simulink model "CornerDetectionHDL_Matlab_Default"  (R2017b)
settings: Solver=FixedStepDiscrete  StartTime=0.0  StopTime=simTime  RelTol=1e-3
InitFcn:
  | % block settings for 240p, change format as appropriate
  | frm2pix = visionhdl.FrameToPixels;
  | frm2pix.VideoFormat = '240p';
  | [activePixelsPerLine, activeLines, totalPixels] = getparamfromfrm2pix(frm2pix);
  | numFrames = 100;
  | simTime = numFrames;
  | % pixel control bus
  | evalin('base','pixelcontrolbus');
undefined symbols (not defined in the file): fspecial, gray, Rec, SDTV
libraries: visionhdlfilter x5, simulink x3, visionhdlio x2, visionconversions x1, visionanalysis x1, visionhdlutilities x1, visionhdlconversions x1, visionhdlmisc x1
settings Model: DataTypeOverride=Off  Creator=The MathWorks, Inc.  LastModifiedBy=KAU-Sprinter
settings DataIOCC: LimitDataPoints=on  SaveFormat=Array  SaveOutput=off  SignalLogging=off  SaveTime=off
settings OptimizationCC: BlockReduction=off  ConditionallyExecuteInputs=off  DefaultParameterBehavior=Inlined  LifeSpan=inf
settings DebuggingCC: AlgebraicLoopMsg=error  ArtificialAlgebraicLoopMsg=none  SingleTaskRateTransMsg=error  IntegerOverflowMsg=none  ParameterPrecisionLossMsg=none  AllowSymbolicDim=off  StrictBusMsg=ErrorOnBusTreatedAsVector  SFUnexpectedBacktrackingDiag=warning  SFNoUnconditionalDefaultTransitionDiag=warning  SFExecutionAtInitializationDiag=none  IntegerSaturationMsg=none
settings HardwareCC: ProdBitPerPointer=32  ProdBitPerSizeT=32  ProdBitPerPtrDiffT=32  ProdLargestAtomicFloat=None  ProdIntDivRoundTo=Undefined  ProdEndianess=Unspecified  ProdWordSize=32  ProdHWDeviceType=ASIC/FPGA->ASIC/FPGA  ProdEqTarget=off
settings ModelReferenceCC: PropagateSignalLabelsOutOfModel=off
settings CodeAppCC: StateflowObjectComments=on
settings GRTTargetCC: TargetLangStandard=C89/C90 (ANSI)  GeneratePreprocessorConditionals=Disable all
settings ConfigComp: CovMetricSettings=dw  CovHtmlReporting=on  CovSaveCumulativeToWorkspaceVar=on  CovSaveSingleToWorkspaceVar=on  CovExternalEMLEnable=off  CovSFcnEnable=off

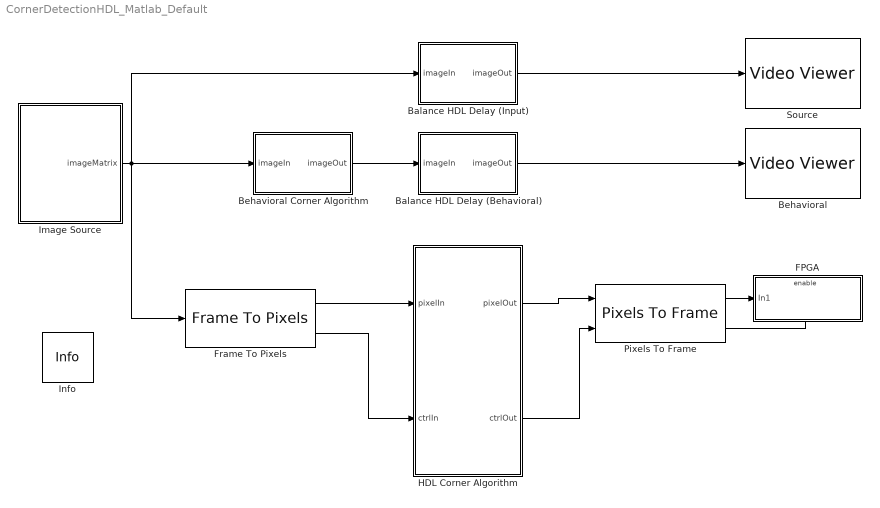
== system CornerDetectionHDL_Matlab_Default ==
  Balance HDL Delay (Behavioral) : Subsystem
  Balance HDL Delay (Input) : Subsystem
  Behavioral : VideoViewer  FigPos=[400.2 479.6 410.4 300]
  Behavioral Corner Algorithm : Subsystem
  FPGA : Subsystem
  Frame To Pixels : visionhdlio/Frame To Pixels  NumComponents=3  VideoFormat=240p  ActivePixelsPerLine=32  ActiveVideoLines=18  TotalPixelsPerLine=42  TotalVideoLines=28  StartingActiveLine=6  FrontPorch=5  SampleTime=0
      settings: SourceProductName=Vision HDL Toolbox  SourceProductBaseCode=VT
  HDL Corner Algorithm : Subsystem  TreatAsAtomicUnit=on
  Image Source : Subsystem  mask(Panning Video Source){VideoFormat=240p}
      mask prompts: VideoFormat "Video Format"
      mask TypeOptions VideoFormat: 240p | 480p | 1080p | Custom
      mask Callback VideoFormat:
      | blk = gcb;
      | set_param(blk,'MaskSelfModifiable','on');
      | maskStr = get_param(blk,'MaskValues');
      | 
      | if strcmpi(maskStr{1},'Custom')
      |     set_param([blk,'/Lines'],'Value',sprintf('[1:%d]',18));
      |     set_param([blk,'/Pixels'],'Value',sprintf('[1:%d]',32));
      | elseif strcmpi(maskStr{1},'240p')
      |     set_param([blk,'/Lines'],'Value',sprintf('[1:%d]',240));
      |     set_param([blk,'/Pixels'],'Value',sprintf('[1:%d]',320));
      | elseif strcmpi(maskStr{1},'480p')
      |     set_param([blk,'/Lines'],'Value',sprintf('[1:%d]',480));
      |     set_param([blk,'/Pixels'],'Value',sprintf('[1:%d]',640));
      | else
      |     set_param([blk,'/Lines'],'Value',sprintf('[1:%d]',1080));
      |     set_param([blk,'/Pixels'],'Value',sprintf('[1:%d]',1920));
      | end
      mask Display: image('cornerboxes.png')
  Info : visionhdlmisc/Info  SystemSampleTime=-1
      settings: SourceProductName=Vision HDL Toolbox  SourceProductBaseCode=VT
  Pixels To Frame : visionhdlio/Pixels To Frame  NumComponents=3  VideoFormat=240p  ActivePixelsPerLine=32  ActiveVideoLines=18  TotalPixelsPerLine=42  TotalVideoLines=28
      settings: SourceProductName=Vision HDL Toolbox  SourceProductBaseCode=VT
  Source : VideoViewer  FigPos=[12.2 436.4 409.6 300]
  wires:
  Image Source/1(imageMatrix) -> Balance HDL Delay (Input)/1(imageIn), Frame To Pixels/1, Behavioral Corner Algorithm/1(imageIn)
  Behavioral Corner Algorithm/1(imageOut) -> Balance HDL Delay (Behavioral)/1(imageIn)
  Frame To Pixels/1 -> HDL Corner Algorithm/1(pixelIn)
  Frame To Pixels/2 -> HDL Corner Algorithm/2(ctrlIn)
  Pixels To Frame/2 -> FPGA/Enable
  Pixels To Frame/1 -> FPGA/1(In1)
  HDL Corner Algorithm/1(pixelOut) -> Pixels To Frame/1
  HDL Corner Algorithm/2(ctrlOut) -> Pixels To Frame/2
  Balance HDL Delay (Input)/1(imageOut) -> Source/1
  Balance HDL Delay (Behavioral)/1(imageOut) -> Behavioral/1

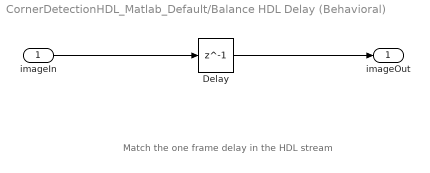
== system CornerDetectionHDL_Matlab_Default/Balance HDL Delay (Behavioral) ==
  note: Match the one frame delay in the HDL stream
  imageIn : Inport
  Delay : Delay  DelayLength=1
  imageOut : Outport
  wires:
  Delay/1 -> imageOut/1
  imageIn/1 -> Delay/1

== system CornerDetectionHDL_Matlab_Default/Balance HDL Delay (Input) ==
  note: Match the one frame delay in the HDL stream
  imageIn : Inport
  Delay : Delay  DelayLength=1
  imageOut : Outport
  wires:
  imageIn/1 -> Delay/1
  Delay/1 -> imageOut/1

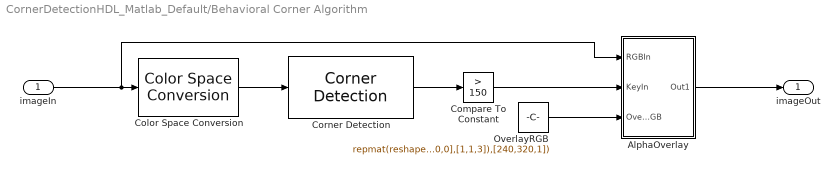
== system CornerDetectionHDL_Matlab_Default/Behavioral Corner Algorithm ==
  imageIn : Inport
  AlphaOverlay : Subsystem
  Color Space Conversion : visionconversions/Color Space  Conversion  conversion=Obsolete  conversionActive=R'G'B' to intensity  wp_str=D65  rec=Rec. 601 (SDTV)  sys=1125/60/2:1  imagePorts=One multidimensional signal
      settings: SourceProductName=Computer Vision System Toolbox
  Compare To Constant : simulink/Logic and Bit Operations/Compare To Constant  relop=>  const=150  OutDataTypeStr=boolean
  Corner Detection : visionanalysis/Corner Detection  method=Harris corner detection (Harris & Stephens)  factor=0.04  filter=fspecial('gaussian', [1 5], 1.5)  thrInten=0.1  thrAngle=157.5  output=Obsolete9b  outputInUse=Metric matrix  maxNum=200  thrMetric=0.0005  neighborSize=[11 11]  isOutVarDim=on  accumMode=Binary point scaling  accumWordLength=32  accumFracLength=0  prodOutputMode=Binary point scaling  prodOutputWordLength=32  prodOutputFracLength=0  memoryMode=Binary point scaling  memoryWordLength=32  memoryFracLength=0  firstCoeffMode=Specify word length  firstCoeffWordLength=16  firstCoeffFracLength=16  roundingMode=Floor  overflowMode=off
      settings: SourceProductName=Computer Vision System Toolbox  SourceProductBaseCode=VP
  "OverlayRGB " : Constant  Value=repmat(reshape([255,0,0],[1,1,3]),[240,320,1])  OutDataTypeStr=uint8
  imageOut : Outport
  wires:
  imageIn/1 -> AlphaOverlay/1(RGBIn), Color Space Conversion/1
  Corner Detection/1 -> Compare To Constant/1
  Color Space Conversion/1 -> Corner Detection/1
  Compare To Constant/1 -> AlphaOverlay/2(KeyIn)
  AlphaOverlay/1(Out1) -> imageOut/1
  "OverlayRGB "/1 -> AlphaOverlay/3(OverlayRGB)

== system CornerDetectionHDL_Matlab_Default/FPGA ==
  In1 : Inport
  Enable : EnablePort
  FPGA Video : VideoViewer  colormapValue=gray(256)  FigPos=[864.2 436.4 416 298.4]
  wires:
  In1/1 -> FPGA Video/1

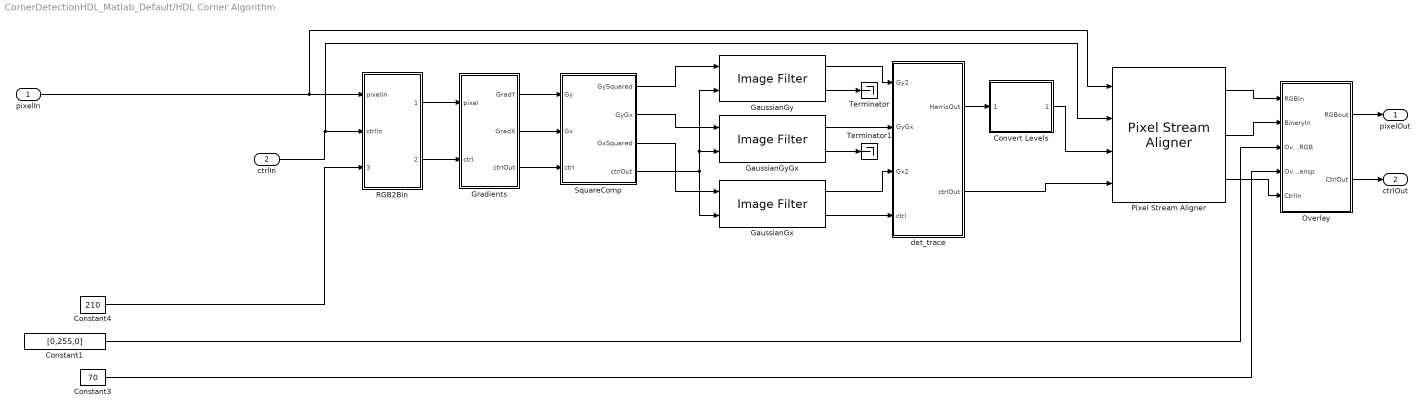
== system CornerDetectionHDL_Matlab_Default/HDL Corner Algorithm ==
  pixelIn : Inport
  ctrlIn : Inport  Port=2
  Constant1 : Constant  Value=[0,255,0]  VectorParams1D=off  OutDataTypeStr=uint8  SampleTime=-1
  Constant3 : Constant  Value=70  OutDataTypeStr=uint8  SampleTime=-1
  Constant4 : Constant  Value=210  OutDataTypeStr=uint8  SampleTime=-1
  Convert Levels : Subsystem
  GaussianGx : visionhdlfilter/Image Filter  Coefficients=fspecial('gaussian',[5,5],1.5)  PaddingMethod=Constant  PaddingValue=0  LineBufferSize=2048  SimulateUsing=Code generation  roundingMode=Floor  overflowMode=off  CoeffDataTypeStr=fixdt(1,18,21)  CoeffMin=[]  CoeffMax=[]  OutputMin=[]  OutputMax=[]
      settings: SourceProductName=Vision HDL Toolbox  SourceProductBaseCode=VT
  GaussianGy : visionhdlfilter/Image Filter  Coefficients=fspecial('gaussian',[5,5],1.5)  PaddingMethod=Constant  PaddingValue=0  LineBufferSize=2048  SimulateUsing=Code generation  roundingMode=Floor  overflowMode=off  CoeffDataTypeStr=fixdt(1,18,21)  CoeffMin=[]  CoeffMax=[]  OutputMin=[]  OutputMax=[]
      settings: SourceProductName=Vision HDL Toolbox  SourceProductBaseCode=VT
  GaussianGyGx : visionhdlfilter/Image Filter  Coefficients=fspecial('gaussian',[5,5],1.5)  PaddingMethod=Constant  PaddingValue=0  LineBufferSize=2048  SimulateUsing=Code generation  roundingMode=Floor  overflowMode=off  CoeffDataTypeStr=fixdt(1,18,21)  CoeffMin=[]  CoeffMax=[]  OutputMin=[]  OutputMax=[]
      settings: SourceProductName=Vision HDL Toolbox  SourceProductBaseCode=VT
  Gradients : Subsystem
  Overlay : Subsystem
  Pixel Stream Aligner : visionhdlutilities/Pixel Stream Aligner  LineBufferSize=2048  MaximumNumberOfLines=10  SimulateUsing=Code generation
      settings: SourceProductName=Vision HDL Toolbox  SourceProductBaseCode=VT
  RGB2Bin : Subsystem
  SquareComp : Subsystem
  Terminator : Terminator
  Terminator1 : Terminator
  det_trace : Subsystem
  pixelOut : Outport
  ctrlOut : Outport  Port=2
  wires:
  Constant1/1 -> Overlay/3(OverlayRGB)
  Constant4/1 -> RGB2Bin/3(SliceLevel)
  RGB2Bin/2(ctrlOut) -> Gradients/2(ctrl)
  Overlay/2("CtrlOut ") -> ctrlOut/1
  Convert Levels/1(PixelOut) -> Pixel Stream Aligner/3
  RGB2Bin/1(pixelOut) -> Gradients/1(pixel)
  Overlay/1(RGBout) -> pixelOut/1
  det_trace/1(HarrisOut) -> Convert Levels/1(HarrisIn)
  Constant3/1 -> Overlay/4(OverlayTransp)
  det_trace/2(ctrlOut) -> Pixel Stream Aligner/4
  Gradients/3(ctrlOut) -> SquareComp/3(ctrl)
  Gradients/2(GradX) -> SquareComp/2(Gx)
  Gradients/1(GradY) -> SquareComp/1(Gy)
  ctrlIn/1 -> Pixel Stream Aligner/2, RGB2Bin/2(ctrlIn)
  pixelIn/1 -> Pixel Stream Aligner/1, RGB2Bin/1(pixelIn)
  GaussianGx/2 -> det_trace/4(ctrl)
  GaussianGx/1 -> det_trace/3(Gx2)
  GaussianGyGx/1 -> det_trace/2(GyGx)
  GaussianGy/1 -> det_trace/1(Gy2)
  SquareComp/3(GxSquared) -> GaussianGx/1
  SquareComp/2(GyGx) -> GaussianGyGx/1
  SquareComp/1(GySquared) -> GaussianGy/1
  SquareComp/4(ctrlOut) -> GaussianGx/2, GaussianGy/2, GaussianGyGx/2
  GaussianGyGx/2 -> Terminator1/1
  GaussianGy/2 -> Terminator/1
  Pixel Stream Aligner/1 -> Overlay/1(RGBIn)
  Pixel Stream Aligner/2 -> Overlay/2(BinaryIn)
  Pixel Stream Aligner/3 -> Overlay/5(CtrlIn)

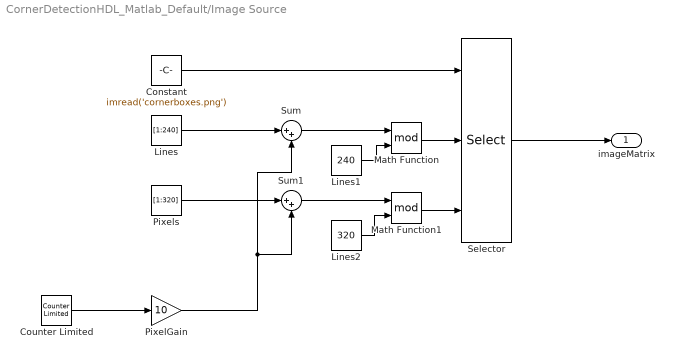
== system CornerDetectionHDL_Matlab_Default/Image Source ==
  Constant : Constant  Value=imread('cornerboxes.png')  VectorParams1D=off
  Counter Limited : simulink/Sources/Counter Limited  uplimit=100  tsamp=1
  Lines : Constant  Value=[1:240]
  Lines1 : Constant  Value=240
  Lines2 : Constant  Value=320
  Math Function : Math  Operator=mod  SaturateOnIntegerOverflow=on
  Math Function1 : Math  Operator=mod  SaturateOnIntegerOverflow=on
  PixelGain : Gain  Gain=10  OutDataTypeStr=double
  Pixels : Constant  Value=[1:320]
  Selector : Selector  NumberOfDimensions=3  IndexMode=Zero-based  InputPortWidth=3  IndexOptions=Index vector (port),Index vector (port),Select all  Indices=[1 3],1,1  OutputSizes=1,1,1
  Sum : Sum  Inputs=|++
  Sum1 : Sum  Inputs=|++
  imageMatrix : Outport
  wires:
  Counter Limited/1 -> PixelGain/1
  Selector/1 -> imageMatrix/1
  Math Function1/1 -> Selector/3
  Constant/1 -> Selector/1
  Math Function/1 -> Selector/2
  Sum/1 -> Math Function/1
  Lines/1 -> Sum/1
  Pixels/1 -> Sum1/1
  PixelGain/1 -> Sum1/2, Sum/2
  Lines1/1 -> Math Function/2
  Lines2/1 -> Math Function1/2
  Sum1/1 -> Math Function1/1

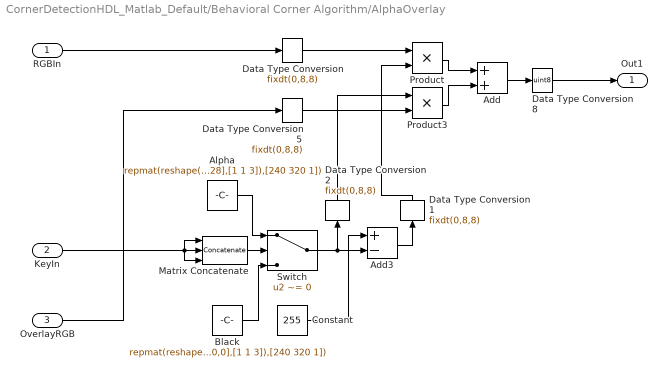
== system CornerDetectionHDL_Matlab_Default/Behavioral Corner Algorithm/AlphaOverlay ==
  RGBIn : Inport
  KeyIn : Inport  Port=2
  OverlayRGB : Inport  Port=3
  Add : Sum  OutDataTypeStr=fixdt(0,8,8)
  Add3 : Sum  Inputs=+-  OutDataTypeStr=uint8
  Alpha : Constant  Value=repmat(reshape([128,128,128],[1 1 3]),[240 320 1])  OutDataTypeStr=uint8
  Black : Constant  Value=repmat(reshape([0,0,0],[1 1 3]),[240 320 1])  OutDataTypeStr=uint8
  Constant : Constant  Value=255  OutDataTypeStr=uint8  SampleTime=-1
  Data Type Conversion{,1..2,5} (4 alike) : DataTypeConversion  OutDataTypeStr=fixdt(0,8,8)  ConvertRealWorld=Stored Integer (SI)
  Data Type Conversion8 : DataTypeConversion  OutDataTypeStr=uint8  ConvertRealWorld=Stored Integer (SI)
  Matrix Concatenate : Concatenate  NumInputs=3  Mode=Multidimensional array  ConcatenateDimension=3
  Product : Product  OutDataTypeStr=fixdt(0,8,8)  SaturateOnIntegerOverflow=on
  Product3 : Product  OutDataTypeStr=fixdt(0,8,8)  SaturateOnIntegerOverflow=on
  Switch : Switch  Criteria=u2 ~= 0
  Out1 : Outport
  wires:
  RGBIn/1 -> Data Type Conversion/1
  Data Type Conversion5/1 -> Product3/2
  Alpha/1 -> Switch/1
  Matrix Concatenate/1 -> Switch/2
  Data Type Conversion2/1 -> Product3/1
  Data Type Conversion1/1 -> Product/2
  KeyIn/1 -> Matrix Concatenate/1, Matrix Concatenate/3, Matrix Concatenate/2
  Data Type Conversion/1 -> Product/1
  Add/1 -> Data Type Conversion8/1
  Product/1 -> Add/1
  Product3/1 -> Add/2
  Data Type Conversion8/1 -> Out1/1
  Black/1 -> Switch/3
  Constant/1 -> Add3/1
  Add3/1 -> Data Type Conversion1/1
  Switch/1 -> Add3/2, Data Type Conversion2/1
  OverlayRGB/1 -> Data Type Conversion5/1

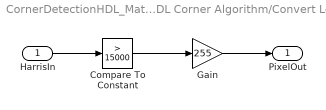
== system CornerDetectionHDL_Matlab_Default/HDL Corner Algorithm/Convert Levels ==
  HarrisIn : Inport
  Compare To Constant : simulink/Logic and Bit Operations/Compare To Constant  relop=>  const=15000  OutDataTypeStr=uint8
  Gain : Gain  Gain=255  OutDataTypeStr=uint8
  PixelOut : Outport
  wires:
  Gain/1 -> PixelOut/1
  HarrisIn/1 -> Compare To Constant/1
  Compare To Constant/1 -> Gain/1

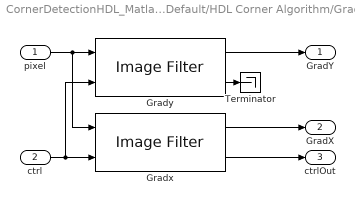
== system CornerDetectionHDL_Matlab_Default/HDL Corner Algorithm/Gradients ==
  pixel : Inport
  ctrl : Inport  Port=2
  Gradx : visionhdlfilter/Image Filter  Coefficients=[0,0,0;1, 0,-1;0,0,0]  PaddingMethod=Replicate  PaddingValue=0  LineBufferSize=2048  SimulateUsing=Code generation  roundingMode=Floor  overflowMode=off  CoeffDataTypeStr=fixdt(1,2,0)  CoeffMin=[]  CoeffMax=[]  OutputDataTypeStr=fixdt(1,9,0)  OutputMin=[]  OutputMax=[]
      settings: SourceProductName=Vision HDL Toolbox  SourceProductBaseCode=VT
  Grady : visionhdlfilter/Image Filter  Coefficients=[0,1,0; 0,0,0; 0,-1,0]  PaddingMethod=Replicate  PaddingValue=0  LineBufferSize=2048  SimulateUsing=Code generation  roundingMode=Floor  overflowMode=off  CoeffDataTypeStr=fixdt(1,2,0)  CoeffMin=[]  CoeffMax=[]  OutputDataTypeStr=fixdt(1,9,0)  OutputMin=[]  OutputMax=[]
      settings: SourceProductName=Vision HDL Toolbox  SourceProductBaseCode=VT
  Terminator : Terminator
  GradY : Outport
  GradX : Outport  Port=2
  ctrlOut : Outport  Port=3
  wires:
  Grady/2 -> Terminator/1
  Gradx/1 -> GradX/1
  Gradx/2 -> ctrlOut/1
  ctrl/1 -> Gradx/2, Grady/2
  pixel/1 -> Grady/1, Gradx/1
  Grady/1 -> GradY/1

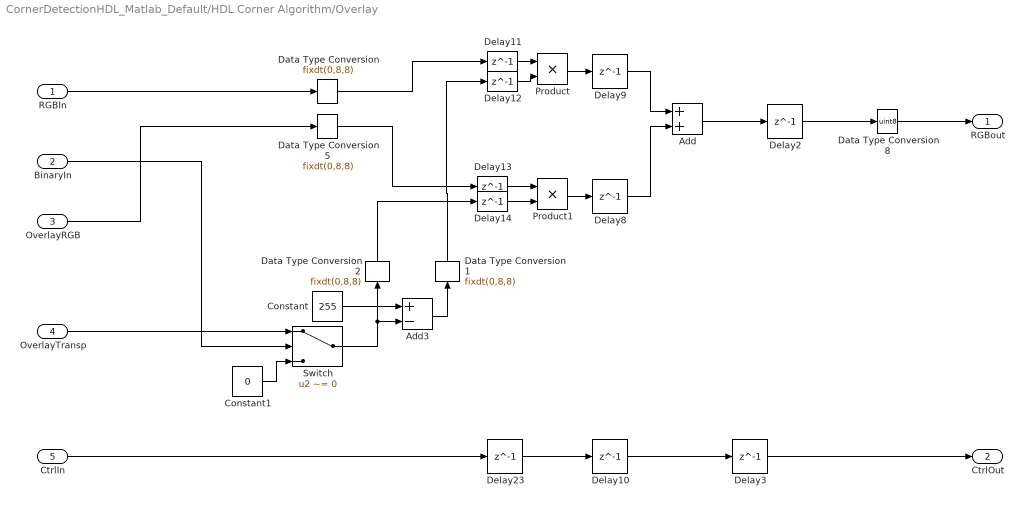
== system CornerDetectionHDL_Matlab_Default/HDL Corner Algorithm/Overlay ==
  RGBIn : Inport
  BinaryIn : Inport  Port=2
  OverlayRGB : Inport  Port=3
  OverlayTransp : Inport  Port=4
  CtrlIn : Inport  Port=5
  Add : Sum  OutDataTypeStr=fixdt(0,8,8)
  Add3 : Sum  Inputs=+-  OutDataTypeStr=uint8
  Constant : Constant  Value=255  OutDataTypeStr=uint8  SampleTime=-1
  Constant1 : Constant  Value=0  OutDataTypeStr=uint8
  Data Type Conversion{,1..2,5} (4 alike) : DataTypeConversion  OutDataTypeStr=fixdt(0,8,8)  ConvertRealWorld=Stored Integer (SI)
  Data Type Conversion8 : DataTypeConversion  OutDataTypeStr=uint8  ConvertRealWorld=Stored Integer (SI)
  Delay{2..3,8..14,23} (10 alike) : Delay  DelayLength=1
  Product : Product  OutDataTypeStr=fixdt(0,8,8)  SaturateOnIntegerOverflow=on
  Product1 : Product  OutDataTypeStr=fixdt(0,8,8)  SaturateOnIntegerOverflow=on
  Switch : Switch  Criteria=u2 ~= 0
  RGBout : Outport
  "CtrlOut " : Outport  Port=2
  wires:
  Add/1 -> Delay2/1
  Constant/1 -> Add3/1
  Add3/1 -> Data Type Conversion1/1
  Switch/1 -> Data Type Conversion2/1, Add3/2
  OverlayTransp/1 -> Switch/1
  BinaryIn/1 -> Switch/2
  Constant1/1 -> Switch/3
  Delay2/1 -> Data Type Conversion8/1
  Delay3/1 -> "CtrlOut "/1
  Product1/1 -> Delay8/1
  Product/1 -> Delay9/1
  Delay9/1 -> Add/1
  Delay8/1 -> Add/2
  Delay10/1 -> Delay3/1
  Delay11/1 -> Product/1
  Delay12/1 -> Product/2
  Delay13/1 -> Product1/1
  Delay14/1 -> Product1/2
  Delay23/1 -> Delay10/1
  CtrlIn/1 -> Delay23/1
  Data Type Conversion/1 -> Delay11/1
  Data Type Conversion1/1 -> Delay12/1
  Data Type Conversion2/1 -> Delay14/1
  OverlayRGB/1 -> Data Type Conversion5/1
  RGBIn/1 -> Data Type Conversion/1
  Data Type Conversion8/1 -> RGBout/1
  Data Type Conversion5/1 -> Delay13/1

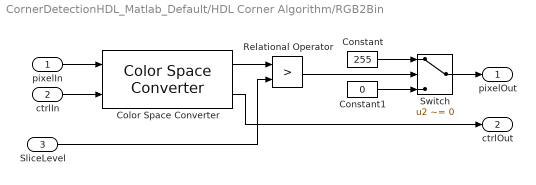
== system CornerDetectionHDL_Matlab_Default/HDL Corner Algorithm/RGB2Bin ==
  pixelIn : Inport
  ctrlIn : Inport  Port=2
  SliceLevel : Inport  Port=3
  Color Space Converter : visionhdlconversions/Color Space Converter  Conversion=RGB to intensity  ConversionStandard=Rec. 601 (SDTV)  ScanningStandard=1250/50/2:1  SimulateUsing=Code generation
      settings: SourceProductName=Vision HDL Toolbox  SourceProductBaseCode=VT
  Constant : Constant  Value=255  OutDataTypeStr=uint8
  Constant1 : Constant  Value=0  OutDataTypeStr=uint8
  Relational Operator : RelationalOperator  Operator=>  OutDataTypeStr=boolean  RndMeth=Nearest
  Switch : Switch  Criteria=u2 ~= 0
  pixelOut : Outport
  ctrlOut : Outport  Port=2
  wires:
  Color Space Converter/2 -> ctrlOut/1
  ctrlIn/1 -> Color Space Converter/2
  pixelIn/1 -> Color Space Converter/1
  Color Space Converter/1 -> Relational Operator/1
  Constant1/1 -> Switch/3
  Constant/1 -> Switch/1
  SliceLevel/1 -> Relational Operator/2
  Relational Operator/1 -> Switch/2
  Switch/1 -> pixelOut/1

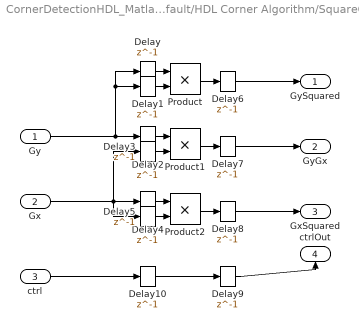
== system CornerDetectionHDL_Matlab_Default/HDL Corner Algorithm/SquareComp ==
  Gy : Inport
  Gx : Inport  Port=2
  ctrl : Inport  Port=3
  Delay{,1..10} (11 alike) : Delay  DelayLength=1  InitialCondition=0
  Product : Product
  Product1 : Product
  Product2 : Product
  GySquared : Outport
  GyGx : Outport  Port=2
  GxSquared : Outport  Port=3
  ctrlOut : Outport  Port=4
  wires:
  Gx/1 -> Delay4/1, Delay5/1, Delay3/1
  Delay5/1 -> Product2/2
  Delay/1 -> Product/1
  Delay1/1 -> Product/2
  Delay2/1 -> Product1/1
  Delay10/1 -> Delay9/1
  Product1/1 -> Delay7/1
  Delay3/1 -> Product1/2
  Product/1 -> Delay6/1
  Product2/1 -> Delay8/1
  Delay4/1 -> Product2/1
  ctrl/1 -> Delay10/1
  Gy/1 -> Delay2/1, Delay/1, Delay1/1
  Delay7/1 -> GyGx/1
  Delay6/1 -> GySquared/1
  Delay8/1 -> GxSquared/1
  Delay9/1 -> ctrlOut/1

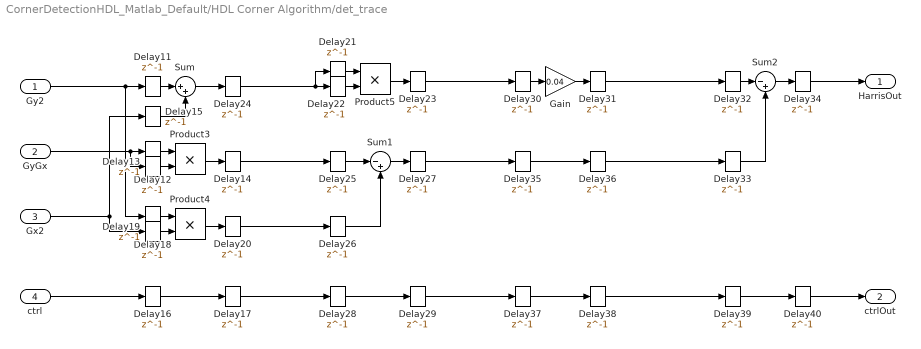
== system CornerDetectionHDL_Matlab_Default/HDL Corner Algorithm/det_trace ==
  Gy2 : Inport
  GyGx : Inport  Port=2
  Gx2 : Inport  Port=3
  ctrl : Inport  Port=4
  Delay{11..40} (30 alike) : Delay  DelayLength=1  InitialCondition=0
  Gain : Gain  Gain=0.04  ParamDataTypeStr=fixdt(0,16,16)  OutDataTypeStr=Inherit: Same as input
  Product3 : Product
  Product4 : Product
  Product5 : Product
  Sum : Sum  Inputs=|++  OutDataTypeStr=Inherit: Same as first input
  Sum1 : Sum  Inputs=|-+
  Sum2 : Sum  Inputs=|-+
  HarrisOut : Outport
  ctrlOut : Outport  Port=2
  wires:
  Delay33/1 -> Sum2/2
  Gain/1 -> Delay31/1
  Delay16/1 -> Delay17/1
  Delay29/1 -> Delay37/1
  Delay23/1 -> Delay30/1
  Delay40/1 -> ctrlOut/1
  Gy2/1 -> Delay11/1, Delay18/1
  Delay36/1 -> Delay33/1
  Delay37/1 -> Delay38/1
  Sum2/1 -> Delay34/1
  Product4/1 -> Delay20/1
  Delay18/1 -> Product4/1
  Delay32/1 -> Sum2/1
  Delay24/1 -> Delay22/1, Delay21/1
  Delay19/1 -> Product4/2
  Delay14/1 -> Delay25/1
  Sum/1 -> Delay24/1
  Delay35/1 -> Delay36/1
  Delay17/1 -> Delay28/1
  Delay28/1 -> Delay29/1
  GyGx/1 -> Delay12/1, Delay13/1
  Delay27/1 -> Delay35/1
  Delay22/1 -> Product5/2
  Delay34/1 -> HarrisOut/1
  Delay20/1 -> Delay26/1
  Delay39/1 -> Delay40/1
  Delay30/1 -> Gain/1
  Delay21/1 -> Product5/1
  Delay38/1 -> Delay39/1
  Delay25/1 -> Sum1/1
  Sum1/1 -> Delay27/1
  Delay26/1 -> Sum1/2
  Delay11/1 -> Sum/1
  Delay13/1 -> Product3/2
  Product5/1 -> Delay23/1
  ctrl/1 -> Delay16/1
  Delay15/1 -> Sum/2
  Delay12/1 -> Product3/1
  Gx2/1 -> Delay15/1, Delay19/1
  Delay31/1 -> Delay32/1
  Product3/1 -> Delay14/1
